simulink model "w1p2"  (R2020b)
settings: Solver=VariableStepAuto  StartTime=0.0  StopTime=10.0  RelTol=1e-3
settings Model: Creator=WELCOME  LastModifiedBy=WELCOME

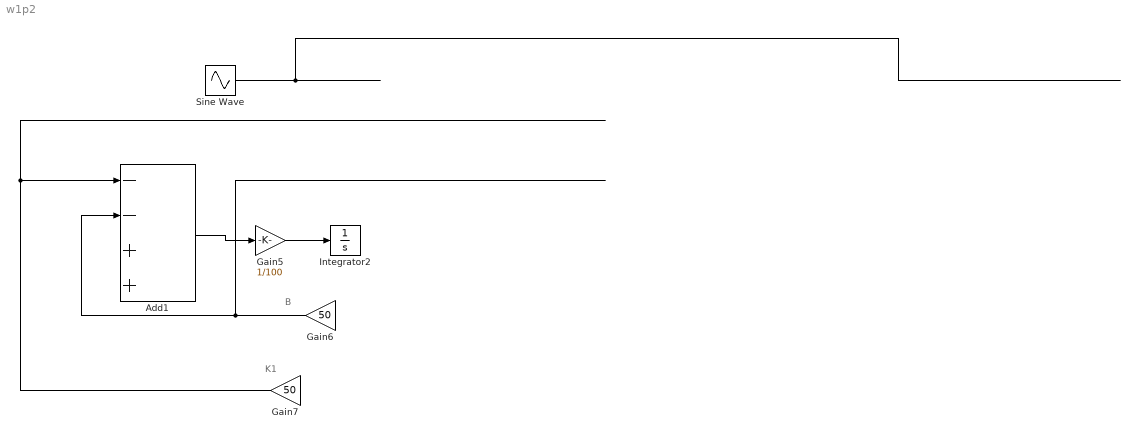
== system w1p2 ==
  note: K1
  note: B
  Add1 : Sum  Inputs=--++
  Gain5 : Gain  Gain=1/100
  Gain6 : Gain  Gain=50
  Gain7 : Gain  Gain=50
  Integrator2 : Integrator
  Sine Wave : Sin  SampleTime=0
  wires:
  ? -> Add1/4
  ? -> Gain7/1
  Gain5/1 -> Integrator2/1
  ? -> Add1/3
  Gain6/1 -> Add1/2
  Sine Wave/1 -> ?
  Gain7/1 -> Add1/1
  Add1/1 -> Gain5/1
  ? -> Gain6/1
